simulink model "Simulation"  (R2024b)
settings: Solver=FixedStepAuto  StartTime=0.0  StopTime=tstop  FixedStep=Time_step  RelTol=1e-3
values from neighbouring files (symbols this model uses):
  BatterySize = BatterySize_new*Energy_convert_sim    (= 10000)    [Auto_preproccesing_energy.m]    (also in preproccesing_energy.m)
  Energy_CombustMax = EnergyMass_Combust*m_dot_CombustMax      *Energy_convert_sim    (= 3606.93)    [Auto_preproccesing_energy.m]    (also in preproccesing_energy.m = 16749.66)
  EnergyMass_Combust = 1.35    [Auto_preproccesing_energy.m]    (also in preproccesing_energy.m = 0.8524)
  m_dot_Reduc = m_Reduc/(5*60)*Time_step    (= 8.2572)    [Auto_preproccesing_energy.m]    (also in preproccesing_energy.m = 3.66666666667)
  Power_Reduc = Energy_Reduc/(5*60)*Time_step      *Energy_convert_sim    (= 1946)    [Auto_preproccesing_energy.m]    (also in preproccesing_energy.m = 1766.66666667)
  StorageSize = StorageSize_new    (= 4000000)    [Auto_preproccesing_energy.m]    (also in preproccesing_energy.m)
settings Model: Creator=20233586  LastModifiedBy=20233586

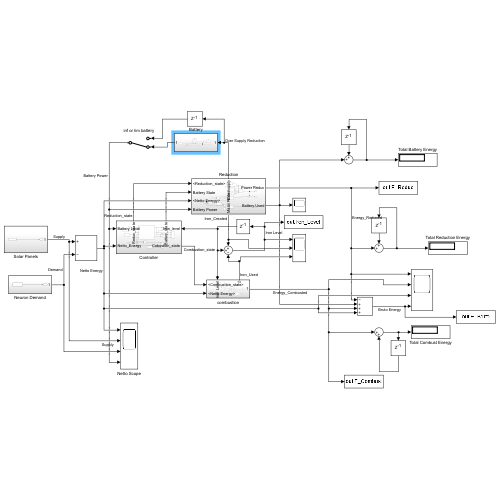
[thumbnail: Simulink's stored preview of the top-level diagram]
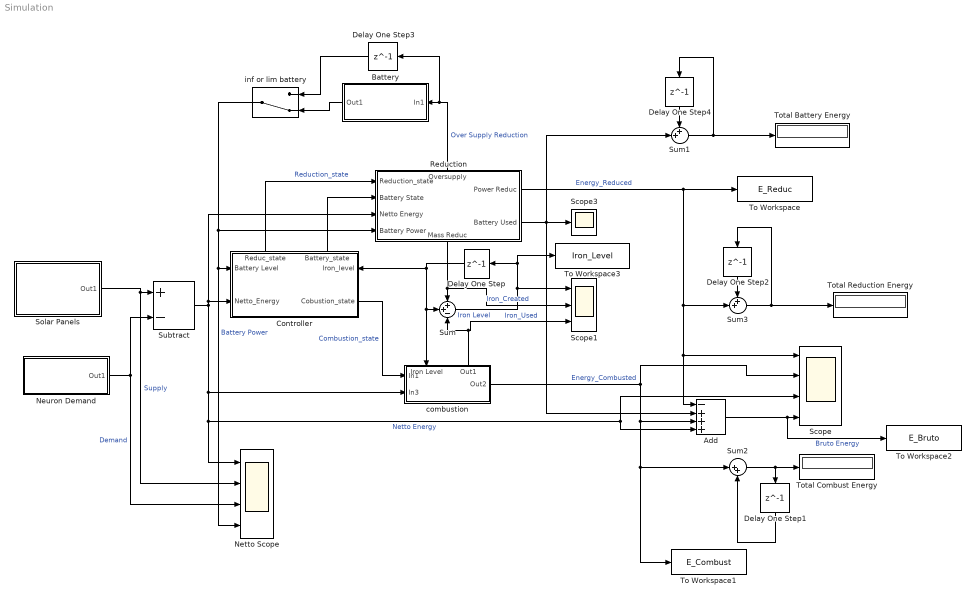
== system Simulation ==
  Add : Sum  Inputs=-+++
  Battery : Subsystem
  Controller : Subsystem
      settings: PortSchema="{\"entries\":[{\"content\":{\"sides\":[{\"content\":{\"connectorIds\":[\"In1\",\"In2\"]},\"type\":\"ConnectorPlacement.EquallySpacedRectSide\",\"uuid\":\"f9190d68-1be9-46bc-b7c1-01b70e76491b\"},{\"content\":{\"connectorIds\":[\"In3\",\"Out1\"],\"side\":\"RIGHT\"},\"type\":\"ConnectorPlacement.EquallySpacedRectSide\",\"uuid\":\"984ed157-bb85-461d-ab0c-9c4d64384457\"},{\"content\":{\"connectorIds\":[\"Out2\",\"Out3\"],\"side\":\"TOP\"},\"type\":\"ConnectorPlacement.EquallySpacedRectSide\",\"uuid\":\"b8c09e09-1b7d-4e7d-abbd-0a35c571f709\"}]},\"type\":\"ConnectorPlacement.EquallySpacedConnector\",\"uuid\":\"02f82c4a-ddad-4528-a200-1a615583cbaa\"}],\"packageUris\":[\"http://schema.mathworks.com/mf0/Connector/R2020b\"],\"version\":\"1.0\"}"
  Delay One Step{,1..4} (5 alike) : Delay  DelayLength=1
  Netto Scope : Scope  NumInputPorts=4
  Neuron Demand : Subsystem
  Reduction : Subsystem
      settings: PortSchema="{\"entries\":[{\"content\":{\"sides\":[{\"content\":{\"connectorIds\":[\"In1\",\"In2\",\"In3\",\"In4\"]},\"type\":\"ConnectorPlacement.EquallySpacedRectSide\",\"uuid\":\"c249e897-8d34-4e7d-972d-5efb6239d870\"},{\"content\":{\"connectorIds\":[\"Out1\",\"Out2\"],\"side\":\"RIGHT\"},\"type\":\"ConnectorPlacement.EquallySpacedRectSide\",\"uuid\":\"6a398f8f-85bb-4775-8de4-b31f61839c68\"},{\"content\":{\"connectorIds\":[\"Out4\"],\"side\":\"TOP\"},\"type\":\"ConnectorPlacement.EquallySpacedRectSide\",\"uuid\":\"7bf51462-98c9-4171-ade8-e3003330355c\"},{\"content\":{\"connectorIds\":[\"Out3\"],\"side\":\"BOTTOM\"},\"type\":\"ConnectorPlacement.EquallySpacedRectSide\",\"uuid\":\"2b09aeff-b1c8-4ca0-baba-0f92a3f3ff9d\"}]},\"type\":\"ConnectorPlacement.EquallySpacedConnector\",\"uuid\":\"664d8217-9812-410b-9be2-917ef6a14661\"}],\"packageUris\":[\"http://schema.mathworks.com/mf0/Connector/R2020b\"],\"version\":\"1.0\"}"
  Scope : Scope  NumInputPorts=4
  Scope1 : Scope  NumInputPorts=3
  Scope3 : Scope
  Solar Panels : Subsystem
  Subtract : Sum  Inputs=+-
  Sum : Sum  Inputs=++-
  Sum1 : Sum  Inputs=++|
  Sum2 : Sum  Inputs=|++
  Sum3 : Sum  Inputs=++|
  To Workspace : ToWorkspace  VariableName=E_Reduc  SaveFormat=Timeseries  SampleTime=-1
  To Workspace1 : ToWorkspace  VariableName=E_Combust  SaveFormat=Timeseries  SampleTime=-1
  To Workspace2 : ToWorkspace  VariableName=E_Bruto  SaveFormat=Timeseries  SampleTime=-1
  To Workspace3 : ToWorkspace  VariableName=Iron_Level  SaveFormat=Timeseries  SampleTime=-1
  Total Battery Energy : Display
  Total Combust Energy : Display
  Total Reduction Energy : Display
  combustion : Subsystem
      settings: PortSchema="{\"entries\":[{\"content\":{\"sides\":[{\"content\":{\"connectorIds\":[\"In1\",\"In2\"]},\"type\":\"ConnectorPlacement.EquallySpacedRectSide\",\"uuid\":\"c249e897-8d34-4e7d-972d-5efb6239d870\"},{\"content\":{\"connectorIds\":[\"Out1\"],\"side\":\"RIGHT\"},\"type\":\"ConnectorPlacement.EquallySpacedRectSide\",\"uuid\":\"6a398f8f-85bb-4775-8de4-b31f61839c68\"},{\"content\":{\"connectorIds\":[\"In3\",\"Out2\"],\"side\":\"TOP\"},\"type\":\"ConnectorPlacement.EquallySpacedRectSide\",\"uuid\":\"7bf51462-98c9-4171-ade8-e3003330355c\"}]},\"type\":\"ConnectorPlacement.EquallySpacedConnector\",\"uuid\":\"664d8217-9812-410b-9be2-917ef6a14661\"}],\"packageUris\":[\"http://schema.mathworks.com/mf0/Connector/R2020b\"],\"version\":\"1.0\"}"
  inf or lim battery : ManualSwitch  CurrentSetting=0
  wires:
  Reduction/3(Mass Reduc) -> Scope1/2, Sum/1  "Iron_Created"
  Solar Panels/1(Out1) -> Netto Scope/2, Subtract/1  "Supply"
  Neuron Demand/1(Out1) -> Subtract/2, Netto Scope/3  "Demand"
  Subtract/1 -> Reduction/3(Netto Energy), Controller/2(Netto_Energy), combustion/2(In3), Netto Scope/1, Add/4, Scope/3  "Netto Energy"
  combustion/1(Out2) -> Add/3, To Workspace1/1, Sum2/1, Scope/2  "Energy_Combusted"
  combustion/2(Out1) -> Scope1/3, Sum/3  "Iron_Used"
  Sum/1 -> To Workspace3/1, Delay One Step/1, Scope1/1  "Iron Level"
  Controller/2(Reduc_state) -> Reduction/1(Reduction_state)  "Reduction_state"
  Controller/1(Cobustion_state) -> combustion/1(In1)  "Combustion_state"
  Reduction/1(Power Reduc) -> Add/1, Scope/1, Sum3/2, To Workspace/1  "Energy_Reduced"
  Delay One Step/1 -> combustion/3(Iron Level), Sum/2, Controller/3(Iron_level)
  Add/1 -> To Workspace2/1, Scope/4  "Bruto Energy"
  Sum2/1 -> Delay One Step1/1, Total Combust Energy/1
  Delay One Step1/1 -> Sum2/2
  Sum3/1 -> Total Reduction Energy/1, Delay One Step2/1
  Delay One Step2/1 -> Sum3/1
  Reduction/4(Oversupply) -> Delay One Step3/1, Battery/1(In1)  "Over Supply Reduction"
  Delay One Step3/1 -> inf or lim battery/1
  Battery/1(Out1) -> inf or lim battery/2
  inf or lim battery/1 -> Netto Scope/4, Controller/1(Battery Level), Reduction/4(Battery Power)  "Battery Power"
  Controller/3(Battery_state) -> Reduction/2(Battery State)
  Reduction/2(Battery Used) -> Sum1/2, Scope3/1, Add/2
  Delay One Step4/1 -> Sum1/1
  Sum1/1 -> Total Battery Energy/1, Delay One Step4/1

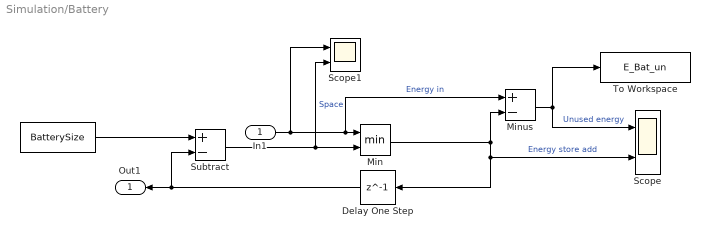
== system Simulation/Battery ==
  In1 : Inport
  " " : Constant  Value=BatterySize
  Delay One Step : Delay  DelayLength=1
  Min : MinMax  Inputs=2
  Minus : Sum  Inputs=+-
  Scope : Scope  NumInputPorts=2
  Scope1 : Scope  NumInputPorts=2
  Subtract : Sum  Inputs=+-
  To Workspace : ToWorkspace  VariableName=E_Bat_un  SaveFormat=Timeseries  SampleTime=-1
  Out1 : Outport
  wires:
  " "/1 -> Subtract/1
  Subtract/1 -> Scope1/2, Min/2  "Space"
  In1/1 -> Scope1/1, Minus/1, Min/1  "Energy in"
  Min/1 -> Delay One Step/1, Scope/2, Minus/2  "Energy store add"
  Minus/1 -> To Workspace/1, Scope/1  "Unused energy"
  Delay One Step/1 -> Out1/1, Subtract/2

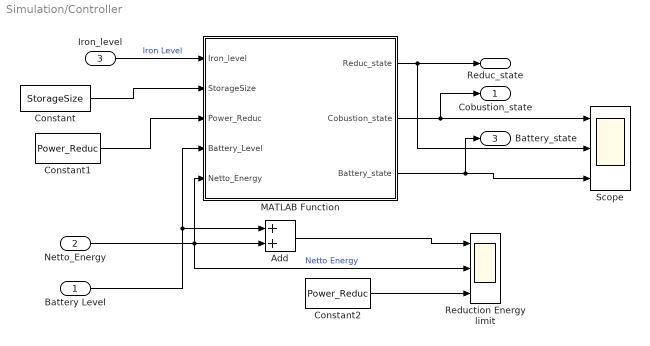
== system Simulation/Controller ==
  Battery Level : Inport
  Netto_Energy : Inport  Port=2
  Iron_level : Inport  Port=3
  Add : Sum
  Constant : Constant  Value=StorageSize
  Constant1 : Constant  Value=Power_Reduc
  Constant2 : Constant  Value=Power_Reduc
  MATLAB Function : MATLAB Function  TreatAsAtomicUnit=on
  Reduction Energy limit : Scope  NumInputPorts=3
  Scope : Scope  NumInputPorts=3
  Cobustion_state : Outport
  Reduc_state : Outport  Port=2
  Battery_state : Outport  Port=3
  wires:
  Iron_level/1 -> MATLAB Function/1(Iron_level)  "Iron Level"
  Netto_Energy/1 -> MATLAB Function/5(Netto_Energy), Add/2, Reduction Energy limit/2  "Netto Energy"
  Constant/1 -> MATLAB Function/2(StorageSize)
  MATLAB Function/2(Cobustion_state) -> Scope/1, Cobustion_state/1
  Constant1/1 -> MATLAB Function/3(Power_Reduc)
  MATLAB Function/1(Reduc_state) -> Reduc_state/1, Scope/2
  Battery Level/1 -> MATLAB Function/4(Battery_Level), Add/1
  MATLAB Function/3(Battery_state) -> Battery_state/1, Scope/3
  Add/1 -> Reduction Energy limit/1
  Constant2/1 -> Reduction Energy limit/3

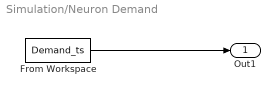
== system Simulation/Neuron Demand ==
  From Workspace : FromWorkspace  VariableName=Demand_ts
  Out1 : Outport
  wires:
  From Workspace/1 -> Out1/1

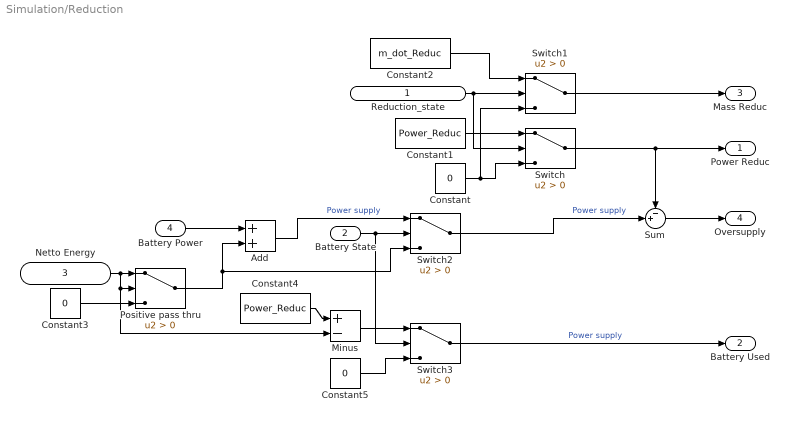
== system Simulation/Reduction ==
  Reduction_state : Inport
  Battery State : Inport  Port=2
  Netto Energy : Inport  Port=3
  Battery Power : Inport  Port=4
  Add : Sum
  Constant : Constant  Value=0
  Constant1 : Constant  Value=Power_Reduc
  Constant2 : Constant  Value=m_dot_Reduc
  Constant3 : Constant  Value=0
  Constant4 : Constant  Value=Power_Reduc
  Constant5 : Constant  Value=0
  Minus : Sum  Inputs=+-
  Positive pass thru : Switch  Criteria=u2 > Threshold  SaturateOnIntegerOverflow=off  InputSameDT=off
  Sum : Sum  Inputs=-+|
  Switch{,1..3} (4 alike) : Switch  Criteria=u2 > Threshold  SaturateOnIntegerOverflow=off  InputSameDT=off
  Power Reduc : Outport
  Battery Used : Outport  Port=2
  Mass Reduc : Outport  Port=3
  Oversupply : Outport  Port=4
  wires:
  Constant2/1 -> Switch1/1
  Reduction_state/1 -> Switch/2, Switch1/2
  Switch/1 -> Sum/1, Power Reduc/1
  Constant/1 -> Switch1/3, Switch/3
  Constant1/1 -> Switch/1
  Switch1/1 -> Mass Reduc/1
  Sum/1 -> Oversupply/1
  Add/1 -> Switch2/1  "Power supply"
  Battery Power/1 -> Add/1
  Switch2/1 -> Sum/2  "Power supply"
  Constant3/1 -> Positive pass thru/3
  Positive pass thru/1 -> Add/2, Switch2/3
  Netto Energy/1 -> Positive pass thru/2, Minus/2, Positive pass thru/1
  Battery State/1 -> Switch3/2, Switch2/2
  Constant5/1 -> Switch3/3
  Constant4/1 -> Minus/1
  Minus/1 -> Switch3/1
  Switch3/1 -> Battery Used/1  "Power supply"

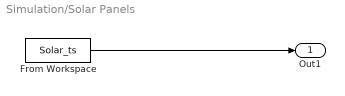
== system Simulation/Solar Panels ==
  From Workspace : FromWorkspace  VariableName=Solar_ts
  Out1 : Outport
  wires:
  From Workspace/1 -> Out1/1

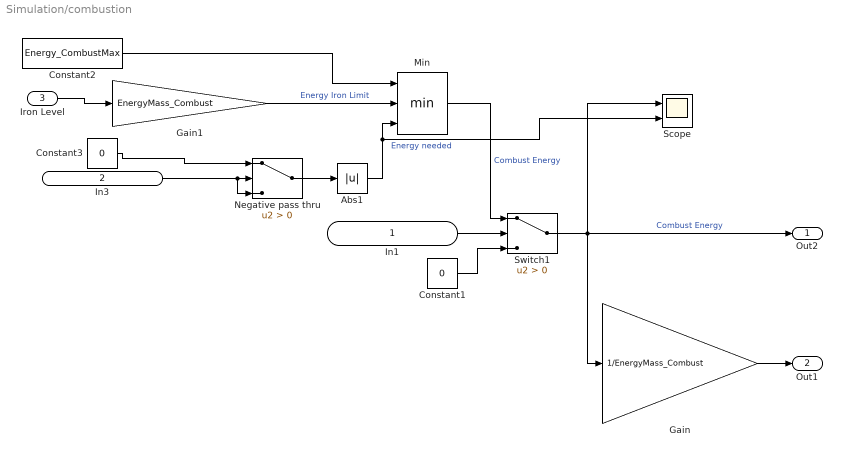
== system Simulation/combustion ==
  In1 : Inport
  In3 : Inport  Port=2
  Iron Level : Inport  Port=3
  Abs1 : Abs  SaturateOnIntegerOverflow=off
  Constant1 : Constant  Value=0
  Constant2 : Constant  Value=Energy_CombustMax
  Constant3 : Constant  Value=0
  Gain : Gain  Gain=1/EnergyMass_Combust
  Gain1 : Gain  Gain=EnergyMass_Combust
  Min : MinMax  Inputs=3
  Negative pass thru : Switch  Criteria=u2 > Threshold  SaturateOnIntegerOverflow=off  InputSameDT=off
  Scope : Scope  NumInputPorts=2
  Switch1 : Switch  Criteria=u2 > Threshold  SaturateOnIntegerOverflow=off  InputSameDT=off
  Out2 : Outport
  Out1 : Outport  Port=2
  wires:
  Gain/1 -> Out1/1
  In1/1 -> Switch1/2
  Constant1/1 -> Switch1/3
  Iron Level/1 -> Gain1/1
  Gain1/1 -> Min/2  "Energy Iron Limit"
  Constant2/1 -> Min/1
  In3/1 -> Negative pass thru/3, Negative pass thru/2
  Constant3/1 -> Negative pass thru/1
  Negative pass thru/1 -> Abs1/1
  Abs1/1 -> Min/3, Scope/2  "Energy needed"
  Switch1/1 -> Scope/1, Out2/1, Gain/1  "Combust Energy"
  Min/1 -> Switch1/1  "Combust Energy"

== matlab function Simulation/Controller/MATLAB Function ==
  data: Iron_level input; StorageSize input; Power_Reduc input; Battery_Level input; Reduc_state output; Netto_Energy input; Cobustion_state output; Battery_state output
function [Reduc_state, Cobustion_state, Battery_state] = fcn(Iron_level, StorageSize, Power_Reduc, Battery_Level, Netto_Energy)

Reduc_state = 0;
Cobustion_state = 0;
Battery_state = 0;

if Iron_level < StorageSize && Netto_Energy > Power_Reduc
    Reduc_state = 1;
elseif Iron_level < StorageSize && Netto_Energy+Battery_Level > Power_Reduc
    Reduc_state = 1;
    Battery_state = 1;
end

if Iron_level > 0 && Netto_Energy < 0
    Cobustion_state = 1;
end
